simulink model "flmpc_simulink"  (R2023a)
settings: Solver=VariableStepAuto  StartTime=0.0  StopTime=inf  RelTol=1e-3
settings Model: Creator=pindiche  LastModifiedBy=pindiche

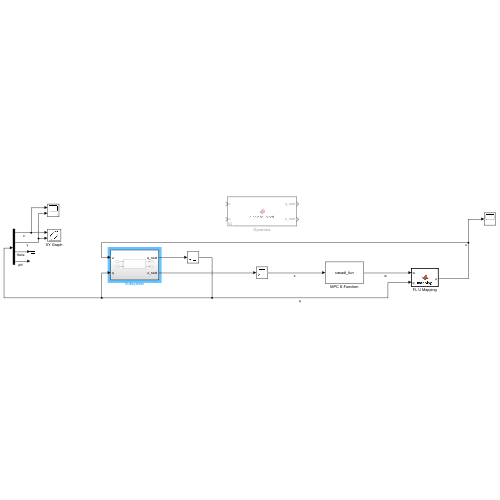
[thumbnail: Simulink's stored preview of the top-level diagram]
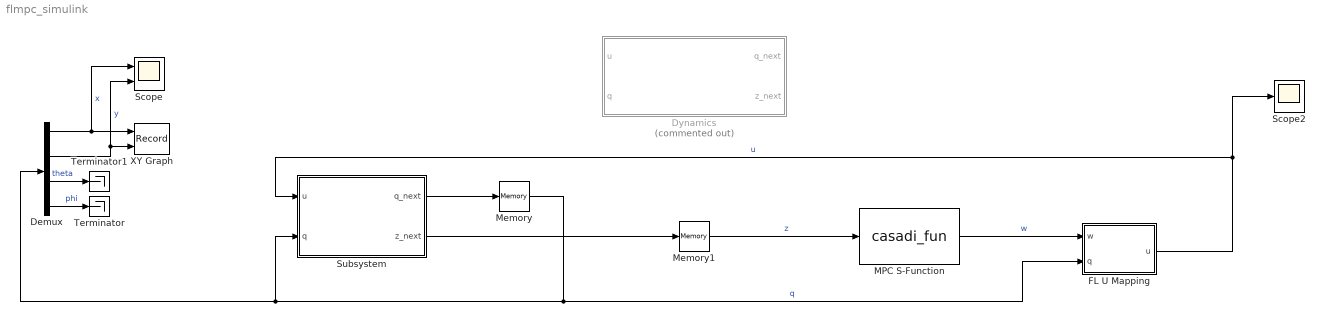
== system flmpc_simulink ==
  Demux : Demux
  Dynamics : MATLAB Function  Commented=on  TreatAsAtomicUnit=on
  FL U Mapping : MATLAB Function  TreatAsAtomicUnit=on
  MPC S-Function : S-Function  FunctionName=casadi_fun  Parameters='flmpc_fun.casadi','flmpc_fun'  SFunctionDeploymentMode=off  EnableBusSupport=off
  Memory : Memory
  Memory1 : Memory
  Scope : Scope  NumInputPorts=2
  Scope2 : Scope
  Subsystem : Subsystem
  Terminator : Terminator
  Terminator1 : Terminator
  XY Graph : Record  FileSettingsInternal="{\"entries\":[{\"content\":{\"excelSettings\":{\"content\":{},\"type\":\"Streamout.ExcelSettings\"}},\"type\":\"Streamout.FileSettingStorage\",\"uuid\":\"\"}],\"packageUris\":[\"http:\\/\\/schema.mathworks.com\\/mf0\\/streamout_blocks\\/R2020a\"],\"version\":\"1.0\"}"  Layout=[1 1]  SignalsInternal="{\"entries\":[{\"content\":{\"signals\":[{\"content\":{\"blockPath\":[],\"dimensions\":[1,1],\"domain\":\"\",\"lineColor\":\"#a2142f\",\"plots\":[1],\"port\":1,\"sid\":[\"\"],\"signalID\":56956,\"signalName\":\"x\"},\"type\":\"RecordBlkView.Signal\",\"uuid\":\"\"},{\"content\":{\"blockPath\":[],\"dimensions\":[1,1],\"domain\":\"\",\"lineColor\":\"#139fff\",\"plots\":[1],\"port\":2,\"sid\":[\"\"],\"signalID\":56960,\"signalName\":\"y\"},\"type\":\"RecordBlkView.Signal\",\"uuid\":\"\"}]},\"type\":\"RecordBlkView.InputSignals\",\"uuid\":\"\"}],\"packageUris\":[\"http:\\/\\/schema.mathworks.com\\/mf0\\/streamout_blocks\\/R2020a\"],\"version\":\"1.0\"}"  VisualizationBindings="{\"xyplotplugin\":{\"info\":[{\"series\":[{\"bindingParametersList\":[{\"parameter\":\"X-Axis\",\"signalID\":56956,\"signalName\":\"x\"},{\"parameter\":\"Y-Axis\",\"signalID\":56960,\"signalName\":\"y\"}],\"seriesID\":13729}],\"subplotID\":1}]}}"  CompatibilityTag=XY
  wires:
  Demux/4 -> Terminator/1  "phi"
  Demux/3 -> Terminator1/1  "theta"
  Demux/1 -> XY Graph/1, Scope/1  "x"
  Demux/2 -> XY Graph/2, Scope/2  "y"
  Memory/1 -> Subsystem/2(q), Demux/1, FL U Mapping/2(q)  "q"
  MPC S-Function/1 -> FL U Mapping/1(w)  "w"
  FL U Mapping/1(u) -> Scope2/1, Subsystem/1(u)  "u"
  Memory1/1 -> MPC S-Function/1  "z"
  Subsystem/1(q_next) -> Memory/1
  Subsystem/2(z_next) -> Memory1/1

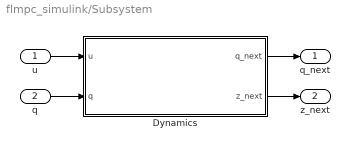
== system flmpc_simulink/Subsystem ==
  u : Inport
  q : Inport  Port=2
  Dynamics : MATLAB Function  TreatAsAtomicUnit=on
  q_next : Outport  PortDimensions=[4,1]
  z_next : Outport  Port=2  PortDimensions=[2,1]
  wires:
  u/1 -> Dynamics/1(u)
  q/1 -> Dynamics/2(q)
  Dynamics/2(z_next) -> z_next/1
  Dynamics/1(q_next) -> q_next/1

== matlab function flmpc_simulink/FL U Mapping ==
  data: w input; u output; q input
function u = mapping(w, q)

Delta = 0.35;
L = 0.256;
eta = [q(3); q(4)];
s1 = sin(eta(1)+eta(2)); c1 = cos(eta(1)+eta(2)); 
M = [cos(eta(1))-tan(eta(2))*(sin(eta(1))+Delta*s1/L), -Delta*s1;
     sin(eta(1))+tan(eta(2))*(cos(eta(1))+Delta*c1/L),  Delta*c1];

u = M^(-1) * w(:, 1);

end

== matlab function flmpc_simulink/Subsystem/Dynamics ==
  data: u input; q_next output; q input; z_next output
function [q_next, z_next] = discrete_plant(u, q)
    % Parameters
    l = 0.256;
    L = l;
    Delta = 0.35;
    dt = 0.1;  
    
    x = q(1);
    y = q(2);
    theta = q(3);
    phi = q(4);
    
    % Extract control inputs
    v = u(1); 
    omega = u(2);  

    % Discretized system dynamics
    x_next = x + dt * (v * cos(theta));  
    y_next = y + dt * (v * sin(theta)); 
    theta_next = theta + dt * (v / l * tan(phi));  
    phi_next = phi + dt * omega; 

    q_next = [x_next; y_next; theta_next; phi_next];
    z_next = [q_next(1)+L*cos(q_next(3))+Delta*cos(q_next(3)+q_next(4));
              q_next(2)+L*sin(q_next(3))+Delta*sin(q_next(3)+q_next(4))];
end

== matlab function flmpc_simulink/Dynamics ==
  data: u input; q_next output; q input; z_next output
function [q_next, z_next] = discrete_plant(u, q)
    % Parameters
    l = 0.256;
    L = l;
    Delta = 0.35;
    dt = 0.1;  
    x = q(1);
    y = q(2);
    theta = q(3);
    phi = q(4);
    
    % Extract control inputs
    v = u(1); 
    omega = u(2);  

    % Discretized system dynamics
    x_next = x + dt * (v * cos(theta));  
    y_next = y + dt * (v * sin(theta)); 
    theta_next = theta + dt * (v / l * tan(phi));  
    phi_next = phi + dt * omega; 

    q_next = [x_next; y_next; theta_next; phi_next];
    z_next = [q_next(1)+L*cos(q_next(3))+Delta*cos(q_next(3)+q_next(4));
              q_next(2)+L*sin(q_next(3))+Delta*sin(q_next(3)+q_next(4))];
end
